simulink model "CSK_FM"  (R2014b)
settings: Solver=ode23s  StartTime=0.0  StopTime=150  RelTol=1e-12
values from neighbouring files (symbols this model uses):
  beta = 25.6    [RUN_021317.m]    (also in RUN_021417.m; RUN_022117.m)
  freq = message baud rate    [ErrChk.m]    (also in LoadText.m = Message Frequency; ProcessSync.m = expected bit frequency; ProcessSyncPeak.m = expected bit frequency; ProcessSyncPeak2.m = expected bit frequency)
  rho = 2    [RUN_021317.m]    (also in RUN_021417.m; RUN_022117.m)
  sig = 10    [RUN_021317.m]    (also in RUN_021417.m; RUN_022117.m)
  x0 = [.1,.2,.3]    [RUN_021317.m]    (also in RUN_021417.m; RUN_022117.m)
libraries: commanapbnd3 x1
settings Model: Creator=Dan  LastModifiedBy=Dan

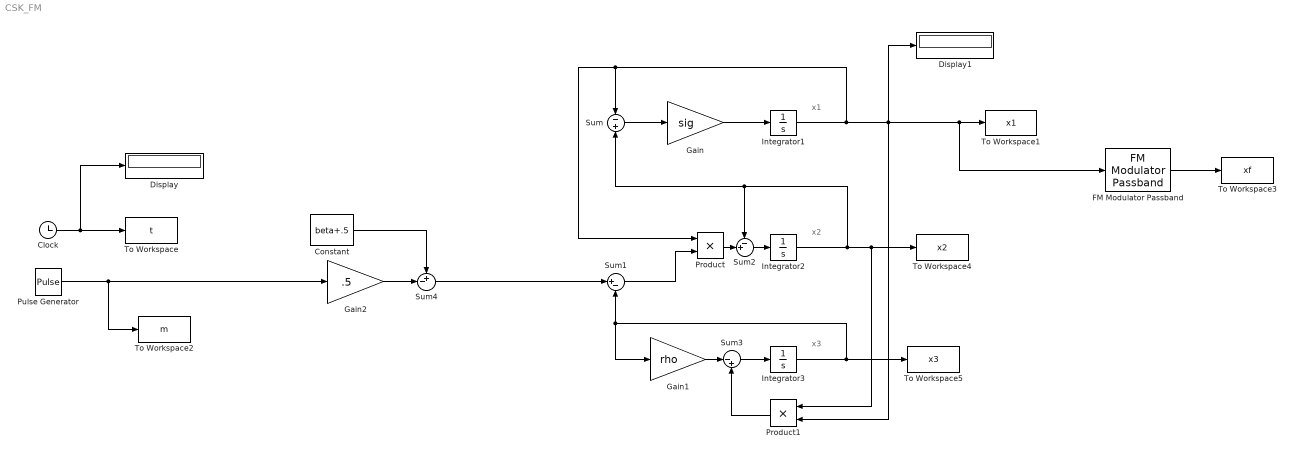
== system CSK_FM ==
  note: x1
  note: x2
  note: x3
  Clock : Clock
  Constant : Constant  Value=beta+.5
  Display : Display
      settings: Decimation=5
  Display1 : Display
      settings: Decimation=5
  FM Modulator Passband : commanapbnd3/FM Modulator Passband  Fc=300  Ph=0  Kc=50
  Gain : Gain  Gain=sig
  Gain1 : Gain  Gain=rho
  Gain2 : Gain  Gain=.5
  Integrator1 : Integrator  InitialCondition=x0(1)
  Integrator2 : Integrator  InitialCondition=x0(2)
  Integrator3 : Integrator  InitialCondition=x0(3)
  Product : Product
  Product1 : Product
  Pulse Generator : DiscretePulseGenerator  PulseType=Time based  Period=2/freq  PulseWidth=50
  Sum : Sum  Inputs=-|+
  Sum1 : Sum  Inputs=|+-
  Sum2 : Sum  Inputs=-+|
  Sum3 : Sum  Inputs=|-+
  Sum4 : Sum  Inputs=+-|
  To Workspace : ToWorkspace  VariableName=t  SampleTime=-1
  To Workspace1 : ToWorkspace  VariableName=x1  SampleTime=-1
  To Workspace2 : ToWorkspace  VariableName=m  SampleTime=-1
  To Workspace3 : ToWorkspace  VariableName=xf  SampleTime=-1
  To Workspace4 : ToWorkspace  VariableName=x2  SampleTime=-1
  To Workspace5 : ToWorkspace  VariableName=x3  SampleTime=-1
  wires:
  Gain/1 -> Integrator1/1
  Sum/1 -> Gain/1
  Sum1/1 -> Product/2
  Integrator3/1 -> To Workspace5/1, Gain1/1, Sum1/2
  Sum3/1 -> Integrator3/1
  Product1/1 -> Sum3/2
  Integrator2/1 -> To Workspace4/1, Product1/1, Sum2/1, Sum/2
  Gain1/1 -> Sum3/1
  Gain2/1 -> Sum4/2
  Constant/1 -> Sum4/1
  Sum4/1 -> Sum1/1
  Clock/1 -> Display/1, To Workspace/1
  Product/1 -> Sum2/2
  Sum2/1 -> Integrator2/1
  Pulse Generator/1 -> To Workspace2/1, Gain2/1
  Integrator1/1 -> Sum/1, Product/1, Product1/2, Display1/1, FM Modulator Passband/1, To Workspace1/1
  FM Modulator Passband/1 -> To Workspace3/1
